simulink model "marine_otter_velocity"  (R2024a)
settings: Solver=FixedStepAuto  StartTime=0.0  StopTime=10.0  FixedStep=0.05  RelTol=1e-3
PostLoadFcn:
  | on_model_load
InitFcn:
  | on_model_start
StopFcn:
  | on_simulation_done
undefined symbols (not defined in the file or in its folder): ActiveScenario
libraries: data_driven_lib_new_ctl x1, marine_lib_sys x1
PostSaveFcn:
  | on_model_save
settings Model: Creator=luka  LastModifiedBy=luka

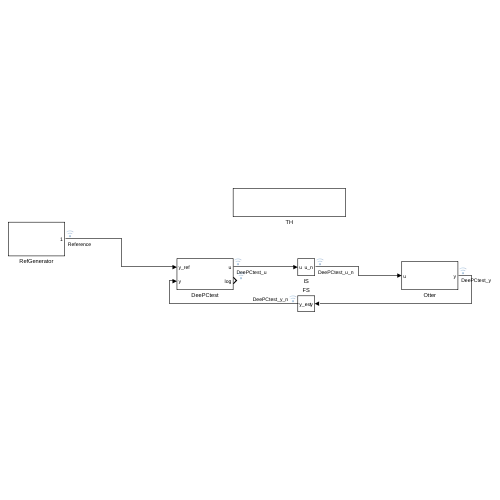
[thumbnail: Simulink's stored preview of the top-level diagram]
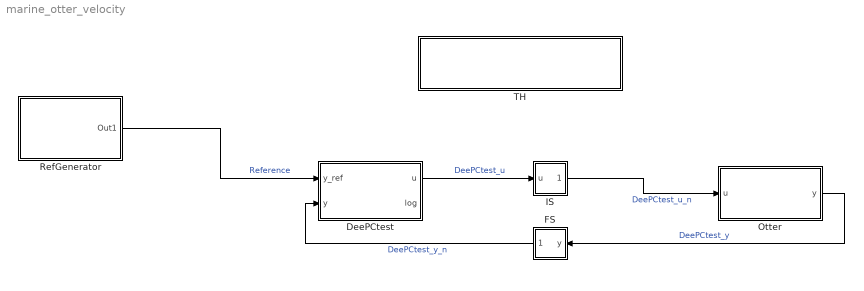
== system marine_otter_velocity ==
  DeePCtest : Subsystem
      mask DialogControl ParameterGroupVar Prompt: Params
  FS : Subsystem
  IS : Subsystem
  Otter : Subsystem
      mask DialogControl ParameterGroupVar Prompt: Params
  RefGenerator : Subsystem  mask{scenario=P1}
      settings: OpenFcn=on_reference_generator_open();
      mask TypeOptions scenario: P1
      mask Callback scenario: on_scenario_select;
  TH : Subsystem
      mask DialogControl ParameterGroupVar Prompt: Params
  wires:
  DeePCtest/1(u) -> IS/1(u)  "DeePCtest_u"
  IS/1(u_n) -> Otter/1(u)  "DeePCtest_u_n"
  Otter/1(y) -> FS/1(y)  "DeePCtest_y"
  FS/1(y_est) -> DeePCtest/2(y)  "DeePCtest_y_n"
  RefGenerator/1(Out1) -> DeePCtest/1(y_ref)  "Reference"

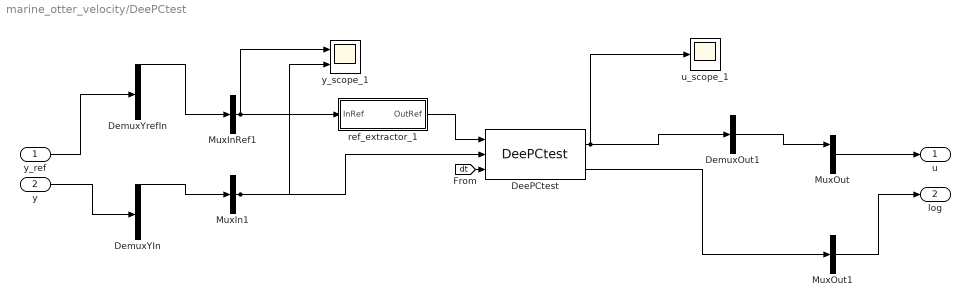
== system marine_otter_velocity/DeePCtest ==
  y_ref : Inport  PortDimensions=12
  y : Inport  Port=2  PortDimensions=12
  DeePCtest : data_driven_lib_new_ctl/DeePCtest  Tag=__cs_comptype:ctl;__cs_compimpl:mat;__cs_casadi;  iid__=[48 99 52 102 55 56 56 101 45 51 56 49 99 45 52 48 49 56 45 57 55 102 52 45 97 102 48 48 102 51 100 57 102 53 53 48]  pid__=[68 101 101 80 67 116 101 115 116 58 100 97 116 97 95 100 114 105 118 101 110 95 108 105 98 95 110 101 119]  params=marine_otter_velocity_params.ctl.DeePCtest  LogEntryType=DeePCtest_LT  cfg_path=cfg_path  data=DeePCtest_data  DataType=DeePCtest_DT  u_ic=0
  DemuxOut1 : Demux  Outputs=1
  DemuxYIn : Demux  Outputs=12
  DemuxYrefIn : Demux  Outputs=12
  MuxIn1 : Mux  Inputs=1
  MuxInRef1 : Mux  Inputs=1
  MuxOut : Mux  Inputs=2
  MuxOut1 : BusCreator  Inputs=1
  ref_extractor_1 : Subsystem
  u_scope_1 : Scope
  y_scope_1 : Scope  NumInputPorts=2
  u : Outport  PortDimensions=2
  log : Outport  Port=2
  wires:
  [dt] -> DeePCtest/3
  y/1 -> DemuxYIn/1
  y_ref/1 -> DemuxYrefIn/1
  MuxOut/1 -> u/1
  MuxOut1/1 -> log/1
  MuxInRef1/1 -> ref_extractor_1/1(InRef), y_scope_1/1
  ref_extractor_1/1(OutRef) -> DeePCtest/1
  MuxIn1/1 -> DeePCtest/2, y_scope_1/2
  DeePCtest/1 -> DemuxOut1/1, u_scope_1/1
  DeePCtest/2 -> MuxOut1/1
  DemuxYIn/1 -> MuxIn1/1
  DemuxYrefIn/1 -> MuxInRef1/1
  DemuxOut1/1 -> MuxOut/1

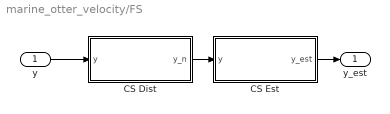
== system marine_otter_velocity/FS ==
  y : Inport
  CS Dist : Subsystem
      mask DialogControl ParameterGroupVar Prompt: Params
  CS Est : Subsystem
      mask DialogControl ParameterGroupVar Prompt: Params
  y_est : Outport
  wires:
  CS Est/1(y_est) -> y_est/1
  CS Dist/1(y_n) -> CS Est/1(y)
  y/1 -> CS Dist/1(y)

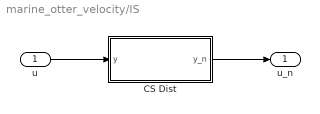
== system marine_otter_velocity/IS ==
  u : Inport
  CS Dist : Subsystem
      mask DialogControl ParameterGroupVar Prompt: Params
  u_n : Outport
  wires:
  CS Dist/1(y_n) -> u_n/1
  u/1 -> CS Dist/1(y)

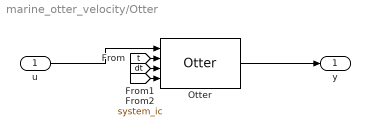
== system marine_otter_velocity/Otter ==
  u : Inport
  Otter : marine_lib_sys/Otter  Tag=system;__cs_slx_sys;__cs_comptype:sys;__cs_compimpl:slx;  payload_mass=0  payload_location=[0,0, 0]  current_speed=0  current_direction=0  out_gain=1  iid__=[52 97 48 100 49 48 49 48 45 52 53 52 57 45 52 100 53 49 45 98 51 97 53 45 54 48 50 101 55 99 57 51 50 98 52 53]  pid__=[79 116 116 101 114 58 109 97 114 105 110 101 95 108 105 98]  params=ActiveScenario.SystemParams  params_struct_name=marine_otter_velocity_params.sys.Otter
  y : Outport
  wires:
  u/1 -> Otter/1
  Otter/1 -> y/1
  [t] -> Otter/2
  [dt] -> Otter/3
  [system_ic] -> Otter/4

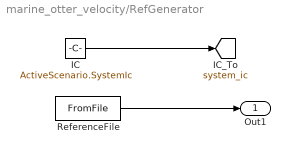
== system marine_otter_velocity/RefGenerator ==
  IC : Constant  Value=ActiveScenario.SystemIc
  ReferenceFile : FromFile  SampleTime=0
  Out1 : Outport
  tag scope: system_ic=global
  wires:
  IC/1 -> [system_ic]
  ReferenceFile/1 -> Out1/1

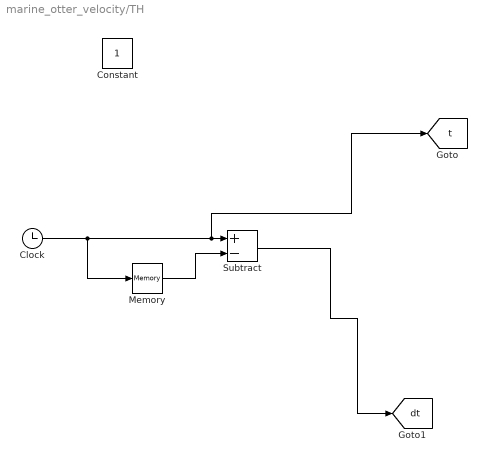
== system marine_otter_velocity/TH ==
  Clock : Clock
  Constant : Constant
  Memory : Memory
  Subtract : Sum  Inputs=+-
  tag scope: dt=global, t=global
  wires:
  Subtract/1 -> [dt]
  Memory/1 -> Subtract/2
  Clock/1 -> Memory/1, Subtract/1, [t]

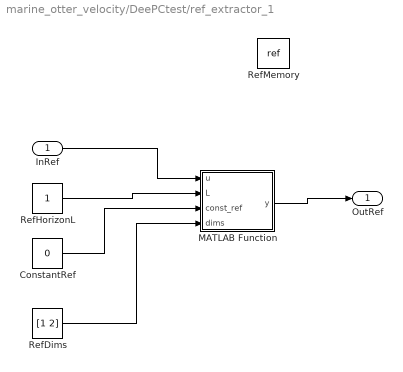
== system marine_otter_velocity/DeePCtest/ref_extractor_1 ==
  InRef : Inport
  ConstantRef : Constant  Value=0
  MATLAB Function : MATLAB Function  TreatAsAtomicUnit=on
  RefDims : Constant  Value=[1 2]
  RefHorizonL : Constant
  RefMemory : DataStoreMemory  DataStoreName=ref  WriteAfterWriteMsg=warning  ShowAdditionalParam=off  OutDataTypeStr=double
  OutRef : Outport
  wires:
  ConstantRef/1 -> MATLAB Function/3(const_ref)
  RefDims/1 -> MATLAB Function/4(dims)
  RefHorizonL/1 -> MATLAB Function/2(L)
  InRef/1 -> MATLAB Function/1(u)
  MATLAB Function/1(y) -> OutRef/1

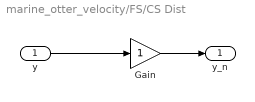
== system marine_otter_velocity/FS/CS Dist ==
  y : Inport
  Gain : Gain
  y_n : Outport
  wires:
  Gain/1 -> y_n/1
  y/1 -> Gain/1

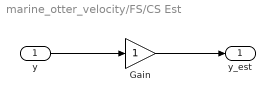
== system marine_otter_velocity/FS/CS Est ==
  y : Inport
  Gain : Gain
  y_est : Outport
  wires:
  y/1 -> Gain/1
  Gain/1 -> y_est/1

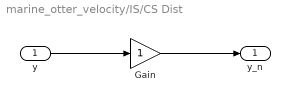
== system marine_otter_velocity/IS/CS Dist ==
  y : Inport
  Gain : Gain
  y_n : Outport
  wires:
  y/1 -> Gain/1
  Gain/1 -> y_n/1

== matlab function marine_otter_velocity/DeePCtest/ref_extractor_1/MATLAB Function ==
  settings: updateMethod=DISCRETE
  data: u input; L input; const_ref input; dims input; y output; ref data_store_memory; GlobalReference parameter
function y = fcn(u, L, const_ref, dims, GlobalReference)

persistent cnt
global ref

if isempty(cnt)
    cnt = 0;
end
cnt = cnt+1;

horizon_end = cnt+L-1;
if L > 1 
   if horizon_end > length(GlobalReference)
        if size(ref, 1) == size(u, 1)
            y = permute(ref, [2, 1]);
        else
            y = ref;
        end       
        return
   end

   if size(ref, 1) == size(u, 1)
      
      if const_ref == 0
        ref(:, :) = GlobalReference(cnt:horizon_end, dims)';
      else
        ref(:, :) = repmat(GlobalReference(cnt, dims)', 1, L);
      end
      y = permute(ref, [2, 1]);
   else
      if const_ref == 0
        ref(1:L, :) = GlobalReference(cnt:horizon_end, dims);
      else
        ref(1:L, :) = repmat(GlobalReference(cnt, dims), L, 1);
      end
      y = ref;
   end
else
   if size(ref, 1) == size(u, 1)
       ref = u;
       y = permute(ref, [2, 1]);
   else
      ref(1, :) = u';
      y = ref;
   end
end
